simulink model "RA2"  (Simulink 8.6)
settings: Solver=ode1  StartTime=0.0  StopTime=1000  FixedStep=1/(1024*4)  RelTol=1e-3
undefined symbols (not defined in the file or in its folder): DiscIntNeverNeededParam
libraries: simulink x4
settings Model: Creator=root  LastModifiedBy=root  SimulationMode=external
settings DataIOCC: LimitDataPoints=off
settings OptimizationCC: InitFltsAndDblsToZero=on
settings DebuggingCC: SolverPrmCheckMsg=none  FcnCallInpInsideContextMsg=UseLocalSettings  UnconnectedInputMsg=none  UnconnectedOutputMsg=none  UnconnectedLineMsg=none  StrictBusMsg=Warning
settings RTWCC: SystemTargetFile=ectarget.tlc  MakeCommand="make_rtw OPTS=\"-DNETIF_ID=2\""  TemplateMakefile=ec_unix.tmf  Description=EtherCAT Real-Time Target for SOEM  RTWVerbose=off
settings GRTTargetCC: UseToolchainInfoCompliant=off  ExtMode=on

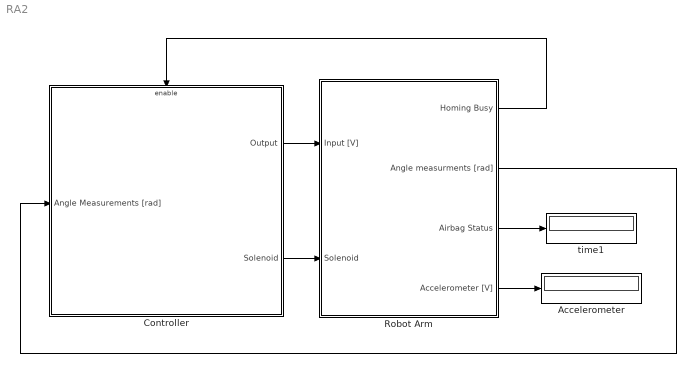
== system RA2 ==
  Accelerometer : Display
      settings: Decimation=50
  Controller : Subsystem
  Robot Arm : Subsystem
      mask help:
      | Robot Arm
      | Hardware: Brom Mechatronica
      | Software: Victor Dolk
      mask Display:
      | image(imread('RobotArm.png'))
      | color('red');port_label('output', 1, 'Homing Busy')
      | port_label('output', 2, 'Angle Measurements')
      | port_label('output', 3, 'Airbag Status')
      | port_label('output', 4, 'Accelerometer [V]')
      | port_label('input', 1, 'Input [V]')
      | port_label('input', 2, 'Solenoid')
  time1 : Display
      settings: Decimation=50
  wires:
  Controller/1(Output) -> Robot Arm/1(Input [V])
  Robot Arm/1(Homing Busy) -> Controller/Enable
  Robot Arm/2(Angle measurments [rad]) -> Controller/1(Angle Measurements [rad])
  Robot Arm/3(Airbag Status) -> time1/1
  Controller/2(Solenoid) -> Robot Arm/2(Solenoid)
  Robot Arm/4(Accelerometer [V]) -> Accelerometer/1

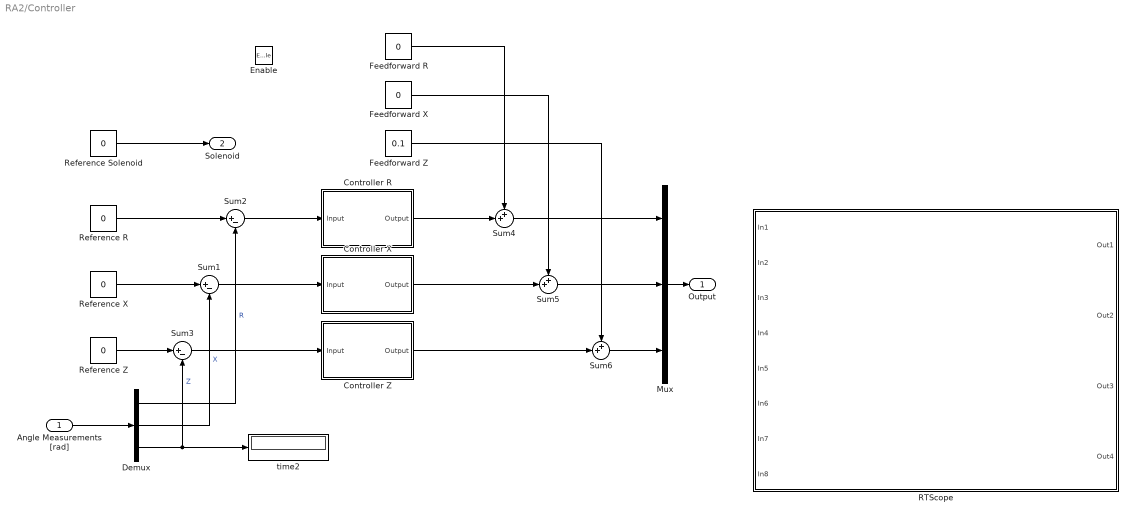
== system RA2/Controller ==
  Angle Measurements [rad] : Inport
  Enable : EnablePort
  Controller R : Subsystem
  Controller X : Subsystem
  Controller Z : Subsystem
  Demux : Demux  Outputs=3
  Feedforward R : Constant  Value=0
  Feedforward X : Constant  Value=0
  Feedforward Z : Constant  Value=0.1
  Mux : Mux  Inputs=3
  RTScope : Subsystem  mask(RTScope){}
      settings: OpenFcn=rtscope
      mask Display: image(imread('rtscope2.jpg'))
  Reference R : Constant  Value=0
  Reference Solenoid : Constant  Value=0
  Reference X : Constant  Value=0
  Reference Z : Constant  Value=0
  Sum1 : Sum  Inputs=|+-
  Sum2 : Sum  Inputs=|+-
  Sum3 : Sum  Inputs=|+-
  Sum4 : Sum  Inputs=++|  SaturateOnIntegerOverflow=on  InputSameDT=on  OutDataTypeStr=Inherit: Same as first input
  Sum5 : Sum  Inputs=++|  SaturateOnIntegerOverflow=on  InputSameDT=on  OutDataTypeStr=Inherit: Same as first input
  Sum6 : Sum  Inputs=++|  SaturateOnIntegerOverflow=on  InputSameDT=on  OutDataTypeStr=Inherit: Same as first input
  time2 : Display
      settings: Decimation=50
  Output : Outport
  Solenoid : Outport  Port=2  InitialOutput=0
  wires:
  Mux/1 -> Output/1
  Angle Measurements [rad]/1 -> Demux/1
  Sum2/1 -> Controller R/1(Input)
  Sum3/1 -> Controller Z/1(Input)
  Sum1/1 -> Controller X/1(Input)
  Demux/1 -> Sum2/2  "R"
  Demux/2 -> Sum1/2  "X"
  Demux/3 -> Sum3/2, time2/1  "Z"
  Feedforward R/1 -> Sum4/1
  Controller R/1(Output) -> Sum4/2
  Sum4/1 -> Mux/1
  Feedforward X/1 -> Sum5/1
  Controller X/1(Output) -> Sum5/2
  Sum5/1 -> Mux/2
  Controller Z/1(Output) -> Sum6/2
  Sum6/1 -> Mux/3
  Feedforward Z/1 -> Sum6/1
  Reference R/1 -> Sum2/1
  Reference X/1 -> Sum1/1
  Reference Z/1 -> Sum3/1
  Reference Solenoid/1 -> Solenoid/1

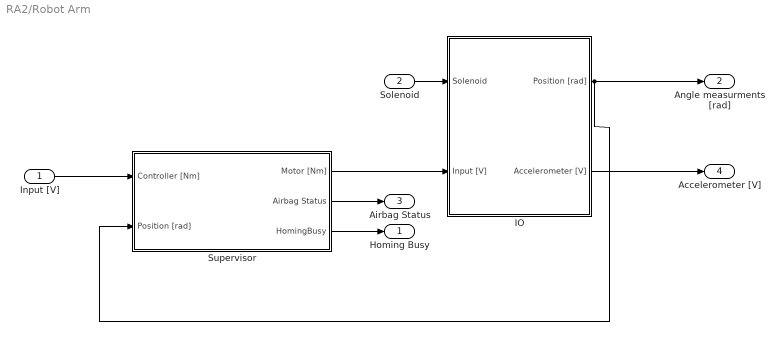
== system RA2/Robot Arm ==
  Input [V] : Inport
  Solenoid : Inport  Port=2
  IO : Subsystem
  Supervisor : Subsystem
  Homing Busy : Outport
  Angle measurments [rad] : Outport  Port=2
  Airbag Status : Outport  Port=3
  Accelerometer [V] : Outport  Port=4
  wires:
  Solenoid/1 -> IO/1(Solenoid)
  Supervisor/1(Motor [Nm]) -> IO/2(Input [V])
  Input [V]/1 -> Supervisor/1(Controller [Nm])
  IO/1(Position [rad]) -> Supervisor/2(Position [rad]), Angle measurments [rad]/1
  Supervisor/2(Airbag Status) -> Airbag Status/1
  Supervisor/3(HomingBusy) -> Homing Busy/1
  IO/2(Accelerometer [V]) -> Accelerometer [V]/1

== system RA2/Controller/Controller R ==
  Input : Inport
  Gain : Gain  Gain=0
  Output : Outport
  wires:
  Input/1 -> Gain/1
  Gain/1 -> Output/1

== system RA2/Controller/Controller X ==
  Input : Inport
  Gain : Gain  Gain=0
  Output : Outport
  wires:
  Gain/1 -> Output/1
  Input/1 -> Gain/1

== system RA2/Controller/Controller Z ==
  Input : Inport
  Gain : Gain  Gain=0
  Output : Outport
  wires:
  Input/1 -> Gain/1
  Gain/1 -> Output/1

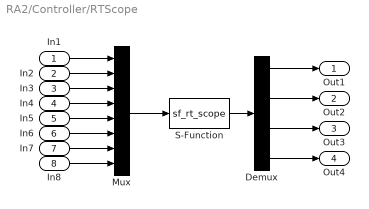
== system RA2/Controller/RTScope ==
  In1 : Inport
  In2 : Inport  Port=2
  In3 : Inport  Port=3
  In4 : Inport  Port=4
  In5 : Inport  Port=5
  In6 : Inport  Port=6
  In7 : Inport  Port=7
  In8 : Inport  Port=8
  Demux : Demux
  Mux : Mux  Inputs=8
  S-Function : S-Function  FunctionName=sf_rt_scope  Parameters=4096  SFunctionDeploymentMode=off  EnableBusSupport=off
  Out1 : Outport
  Out2 : Outport  Port=2
  Out3 : Outport  Port=3
  Out4 : Outport  Port=4
  wires:
  In8/1 -> Mux/8
  In7/1 -> Mux/7
  In6/1 -> Mux/6
  In5/1 -> Mux/5
  In4/1 -> Mux/4
  In3/1 -> Mux/3
  In2/1 -> Mux/2
  In1/1 -> Mux/1
  Demux/4 -> Out4/1
  Demux/3 -> Out3/1
  Demux/2 -> Out2/1
  Demux/1 -> Out1/1
  S-Function/1 -> Demux/1
  Mux/1 -> S-Function/1

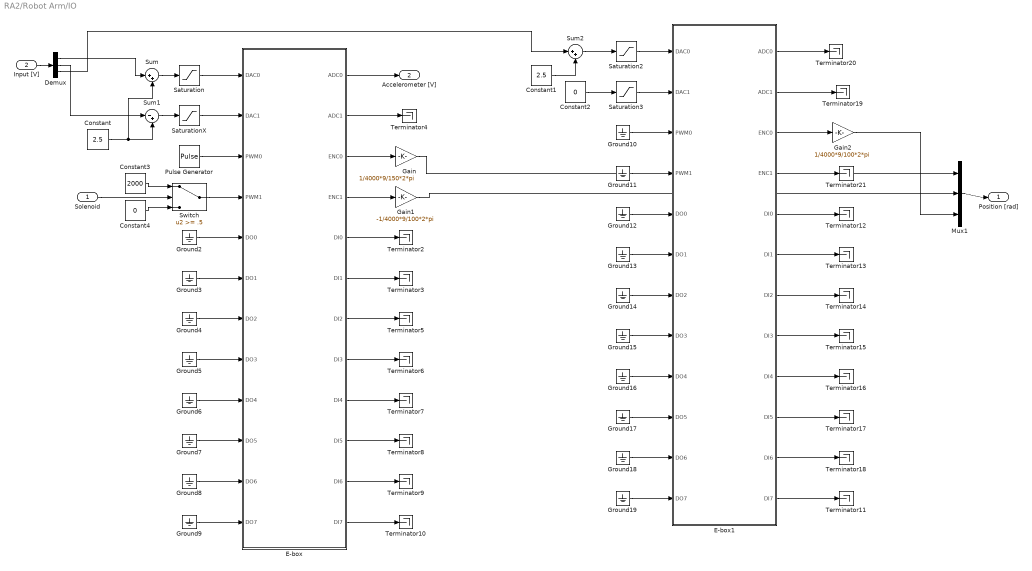
== system RA2/Robot Arm/IO ==
  Solenoid : Inport
  Input [V] : Inport  Port=2
  Constant : Constant  Value=2.5
  Constant1 : Constant  Value=2.5
  Constant2 : Constant  Value=0
  Constant3 : Constant  Value=2000
  Constant4 : Constant  Value=0
  Demux : Demux  Outputs=3
  E-box : Subsystem  mask(E-box){link_id=0}
      mask prompts: link_id "Link id (>=0)"
  E-box1 : Subsystem  mask(E-box){link_id=1}
      mask prompts: link_id "Link id (>=0)"
  Gain : Gain  Gain=1/4000*9/150*2*pi
  Gain1 : Gain  Gain=-1/4000*9/100*2*pi
  Gain2 : Gain  Gain=1/4000*9/100*2*pi
  Ground{2..19} (18 alike) : Ground
  Mux1 : Mux  Inputs=3
  Pulse Generator : DiscretePulseGenerator  PulseType=Time based  Amplitude=2000  Period=1/1024  PulseWidth=50
  Saturation : Saturate  UpperLimit=5  LowerLimit=0
  Saturation2 : Saturate  UpperLimit=5  LowerLimit=0
  Saturation3 : Saturate  UpperLimit=5  LowerLimit=0
  SaturationX : Saturate  UpperLimit=5  LowerLimit=0
  Sum : Sum  Inputs=|++
  Sum1 : Sum  Inputs=|-+
  Sum2 : Sum  Inputs=|++
  Switch : Switch  Threshold=.5
  Terminator{2..21} (20 alike) : Terminator
  Position [rad] : Outport
  Accelerometer [V] : Outport  Port=2
  wires:
  E-box/3(ENC0) -> Gain/1
  Gain/1 -> Mux1/1
  E-box1/3(ENC0) -> Gain2/1
  E-box/4(ENC1) -> Gain1/1
  Saturation/1 -> E-box/1(DAC0)
  SaturationX/1 -> E-box/2(DAC1)
  Saturation2/1 -> E-box1/1(DAC0)
  Saturation3/1 -> E-box1/2(DAC1)
  Ground2/1 -> E-box/5(DO0)
  Ground3/1 -> E-box/6(DO1)
  Ground4/1 -> E-box/7(DO2)
  Ground5/1 -> E-box/8(DO3)
  Ground6/1 -> E-box/9(DO4)
  Ground7/1 -> E-box/10(DO5)
  Ground8/1 -> E-box/11(DO6)
  Ground9/1 -> E-box/12(DO7)
  Ground10/1 -> E-box1/3(PWM0)
  Ground11/1 -> E-box1/4(PWM1)
  Ground12/1 -> E-box1/5(DO0)
  Ground13/1 -> E-box1/6(DO1)
  Ground14/1 -> E-box1/7(DO2)
  Ground15/1 -> E-box1/8(DO3)
  Ground16/1 -> E-box1/9(DO4)
  Ground17/1 -> E-box1/10(DO5)
  Ground18/1 -> E-box1/11(DO6)
  Ground19/1 -> E-box1/12(DO7)
  E-box/12(DI7) -> Terminator10/1
  E-box/11(DI6) -> Terminator9/1
  E-box/10(DI5) -> Terminator8/1
  E-box/9(DI4) -> Terminator7/1
  E-box/8(DI3) -> Terminator6/1
  E-box/7(DI2) -> Terminator5/1
  E-box/6(DI1) -> Terminator3/1
  E-box/5(DI0) -> Terminator2/1
  E-box1/12(DI7) -> Terminator11/1
  E-box1/11(DI6) -> Terminator18/1
  E-box1/10(DI5) -> Terminator17/1
  E-box1/9(DI4) -> Terminator16/1
  E-box1/8(DI3) -> Terminator15/1
  E-box1/7(DI2) -> Terminator14/1
  E-box1/6(DI1) -> Terminator13/1
  E-box1/5(DI0) -> Terminator12/1
  E-box1/2(ADC1) -> Terminator19/1
  E-box1/4(ENC1) -> Terminator21/1
  Constant2/1 -> Saturation3/1
  Gain1/1 -> Mux1/2
  Gain2/1 -> Mux1/3
  Demux/1 -> Sum/1
  Sum/1 -> Saturation/1
  Demux/2 -> Sum1/1
  Constant/1 -> Sum/2, Sum1/2
  Sum2/1 -> Saturation2/1
  Demux/3 -> Sum2/1
  Constant1/1 -> Sum2/2
  Sum1/1 -> SaturationX/1
  E-box/2(ADC1) -> Terminator4/1
  E-box1/1(ADC0) -> Terminator20/1
  Pulse Generator/1 -> E-box/3(PWM0)
  Switch/1 -> E-box/4(PWM1)
  Constant4/1 -> Switch/3
  Constant3/1 -> Switch/1
  Solenoid/1 -> Switch/2
  Input [V]/1 -> Demux/1
  Mux1/1 -> Position [rad]/1
  E-box/1(ADC0) -> Accelerometer [V]/1

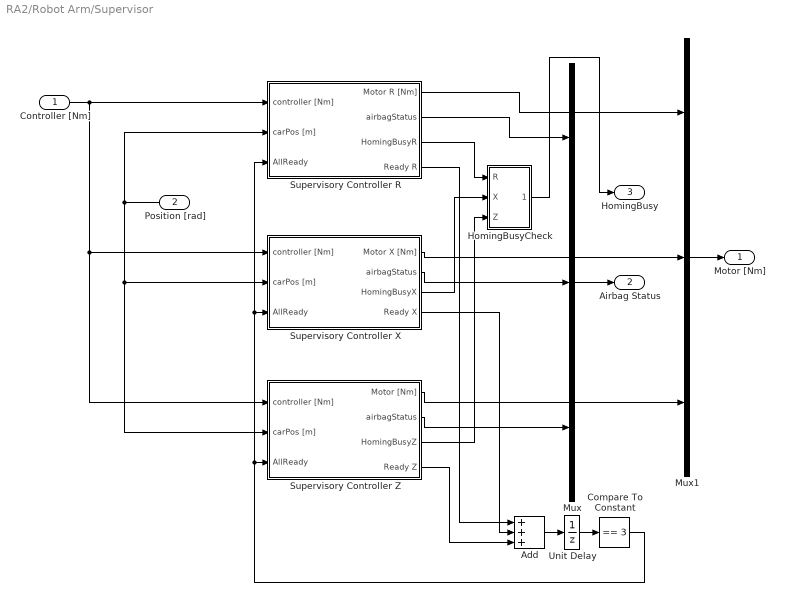
== system RA2/Robot Arm/Supervisor ==
  Controller [Nm] : Inport
  Position [rad] : Inport  Port=2
  Add : Sum  Inputs=+++
  Compare To Constant : simulink/Logic and Bit Operations/Compare To Constant  relop===  const=3  OutDataTypeStr=boolean
  HomingBusyCheck : Subsystem
  Mux : Mux  Inputs=3
  Mux1 : Mux  Inputs=3
  Supervisory Controller R : Subsystem
  Supervisory Controller X : Subsystem
  Supervisory Controller Z : Subsystem
  Unit Delay : UnitDelay  SampleTime=-1
  Motor [Nm] : Outport
  Airbag Status : Outport  Port=2
  HomingBusy : Outport  Port=3
  wires:
  Controller [Nm]/1 -> Supervisory Controller R/1(controller [Nm]), Supervisory Controller X/1(controller [Nm]), Supervisory Controller Z/1(controller [Nm])
  Mux/1 -> Airbag Status/1
  Supervisory Controller R/2(airbagStatus) -> Mux/1
  Supervisory Controller X/2(airbagStatus) -> Mux/2
  Supervisory Controller Z/2(airbagStatus) -> Mux/3
  Supervisory Controller R/1(Motor R [Nm]) -> Mux1/1
  Supervisory Controller X/1(Motor X [Nm]) -> Mux1/2
  Supervisory Controller Z/1(Motor [Nm]) -> Mux1/3
  Position [rad]/1 -> Supervisory Controller R/2(carPos [m]), Supervisory Controller X/2(carPos [m]), Supervisory Controller Z/2(carPos [m])
  Mux1/1 -> Motor [Nm]/1
  Supervisory Controller R/3(HomingBusyR) -> HomingBusyCheck/1(R)
  Supervisory Controller X/3(HomingBusyX) -> HomingBusyCheck/2(X)
  Supervisory Controller Z/3(HomingBusyZ) -> HomingBusyCheck/3(Z)
  HomingBusyCheck/1(Out1) -> HomingBusy/1
  Supervisory Controller R/4(Ready R) -> Add/1
  Supervisory Controller X/4(Ready X) -> Add/2
  Supervisory Controller Z/4(Ready Z) -> Add/3
  Compare To Constant/1 -> Supervisory Controller Z/3(AllReady), Supervisory Controller X/3(AllReady), Supervisory Controller R/3(AllReady)
  Add/1 -> Unit Delay/1
  Unit Delay/1 -> Compare To Constant/1

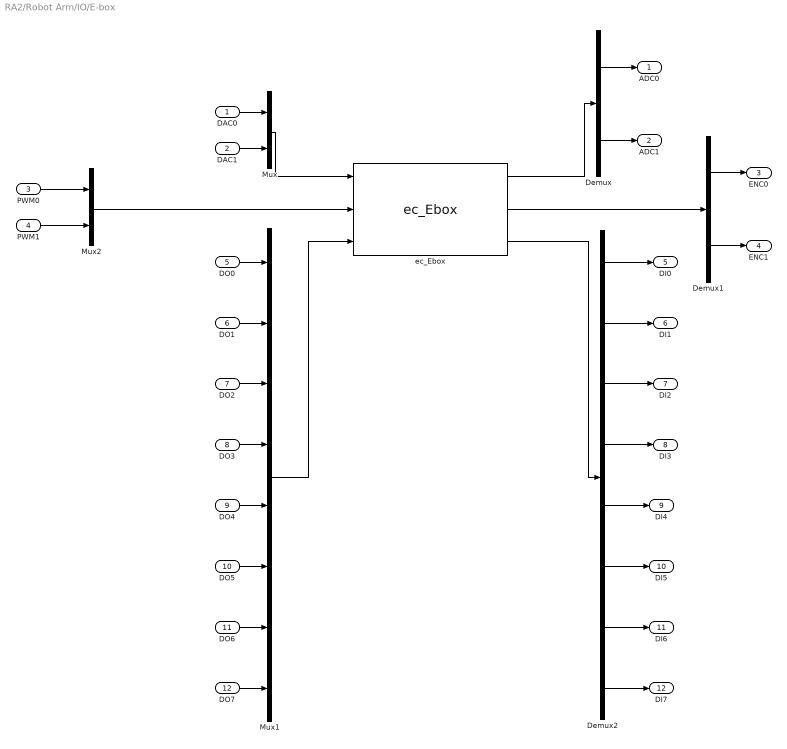
== system RA2/Robot Arm/IO/E-box ==
  DAC0 : Inport
  DAC1 : Inport  Port=2
  PWM0 : Inport  Port=3
  PWM1 : Inport  Port=4
  DO0 : Inport  Port=5
  DO1 : Inport  Port=6
  DO2 : Inport  Port=7
  DO3 : Inport  Port=8
  DO4 : Inport  Port=9
  DO5 : Inport  Port=10
  DO6 : Inport  Port=11
  DO7 : Inport  Port=12
  Demux : Demux  Outputs=2
  Demux1 : Demux  Outputs=2
  Demux2 : Demux  Outputs=8
  Mux : Mux  Inputs=2
  Mux1 : Mux  Inputs=8
  Mux2 : Mux  Inputs=2
  ec_Ebox : S-Function  FunctionName=ec_Ebox  Parameters=link_id  SFunctionDeploymentMode=off  EnableBusSupport=off  mask{link_id=link_id}
      mask prompts: link_id "analog in id (start from 1)"
      mask Display:
      | port_label('output',1,'ADC')
      | port_label('output',2,'ENC')
      | port_label('output',3,'DI')
      | port_label('input',1,'DAC')
      | port_label('input',2,'PWM')
      | port_label('input',3,'DO')
  ADC0 : Outport
  ADC1 : Outport  Port=2
  ENC0 : Outport  Port=3
  ENC1 : Outport  Port=4
  DI0 : Outport  Port=5
  DI1 : Outport  Port=6
  DI2 : Outport  Port=7
  DI3 : Outport  Port=8
  DI4 : Outport  Port=9
  DI5 : Outport  Port=10
  DI6 : Outport  Port=11
  DI7 : Outport  Port=12
  wires:
  ec_Ebox/1 -> Demux/1
  Demux/1 -> ADC0/1
  Demux/2 -> ADC1/1
  Demux1/1 -> ENC0/1
  Demux1/2 -> ENC1/1
  ec_Ebox/2 -> Demux1/1
  Mux/1 -> ec_Ebox/1
  DAC0/1 -> Mux/1
  DAC1/1 -> Mux/2
  ec_Ebox/3 -> Demux2/1
  Demux2/1 -> DI0/1
  Demux2/2 -> DI1/1
  Demux2/3 -> DI2/1
  Demux2/4 -> DI3/1
  Demux2/5 -> DI4/1
  Demux2/6 -> DI5/1
  Demux2/7 -> DI6/1
  Demux2/8 -> DI7/1
  DO0/1 -> Mux1/1
  DO1/1 -> Mux1/2
  DO2/1 -> Mux1/3
  DO3/1 -> Mux1/4
  DO4/1 -> Mux1/5
  DO5/1 -> Mux1/6
  DO6/1 -> Mux1/7
  DO7/1 -> Mux1/8
  Mux1/1 -> ec_Ebox/3
  Mux2/1 -> ec_Ebox/2
  PWM0/1 -> Mux2/1
  PWM1/1 -> Mux2/2

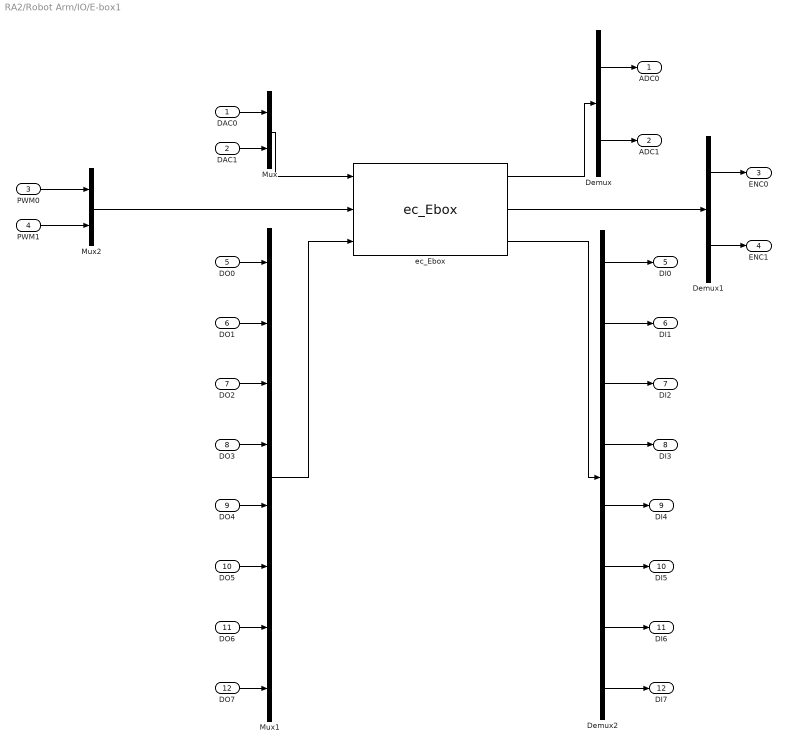
== system RA2/Robot Arm/IO/E-box1 ==
  DAC0 : Inport
  DAC1 : Inport  Port=2
  PWM0 : Inport  Port=3
  PWM1 : Inport  Port=4
  DO0 : Inport  Port=5
  DO1 : Inport  Port=6
  DO2 : Inport  Port=7
  DO3 : Inport  Port=8
  DO4 : Inport  Port=9
  DO5 : Inport  Port=10
  DO6 : Inport  Port=11
  DO7 : Inport  Port=12
  Demux : Demux  Outputs=2
  Demux1 : Demux  Outputs=2
  Demux2 : Demux  Outputs=8
  Mux : Mux  Inputs=2
  Mux1 : Mux  Inputs=8
  Mux2 : Mux  Inputs=2
  ec_Ebox : S-Function  FunctionName=ec_Ebox  Parameters=link_id  SFunctionDeploymentMode=off  EnableBusSupport=off  mask{link_id=link_id}
      mask prompts: link_id "analog in id (start from 1)"
      mask Display:
      | port_label('output',1,'ADC')
      | port_label('output',2,'ENC')
      | port_label('output',3,'DI')
      | port_label('input',1,'DAC')
      | port_label('input',2,'PWM')
      | port_label('input',3,'DO')
  ADC0 : Outport
  ADC1 : Outport  Port=2
  ENC0 : Outport  Port=3
  ENC1 : Outport  Port=4
  DI0 : Outport  Port=5
  DI1 : Outport  Port=6
  DI2 : Outport  Port=7
  DI3 : Outport  Port=8
  DI4 : Outport  Port=9
  DI5 : Outport  Port=10
  DI6 : Outport  Port=11
  DI7 : Outport  Port=12
  wires:
  PWM1/1 -> Mux2/2
  PWM0/1 -> Mux2/1
  Mux2/1 -> ec_Ebox/2
  Mux1/1 -> ec_Ebox/3
  DO7/1 -> Mux1/8
  DO6/1 -> Mux1/7
  DO5/1 -> Mux1/6
  DO4/1 -> Mux1/5
  DO3/1 -> Mux1/4
  DO2/1 -> Mux1/3
  DO1/1 -> Mux1/2
  DO0/1 -> Mux1/1
  Demux2/8 -> DI7/1
  Demux2/7 -> DI6/1
  Demux2/6 -> DI5/1
  Demux2/5 -> DI4/1
  Demux2/4 -> DI3/1
  Demux2/3 -> DI2/1
  Demux2/2 -> DI1/1
  Demux2/1 -> DI0/1
  ec_Ebox/3 -> Demux2/1
  DAC1/1 -> Mux/2
  DAC0/1 -> Mux/1
  Mux/1 -> ec_Ebox/1
  ec_Ebox/2 -> Demux1/1
  Demux1/2 -> ENC1/1
  Demux1/1 -> ENC0/1
  Demux/2 -> ADC1/1
  Demux/1 -> ADC0/1
  ec_Ebox/1 -> Demux/1

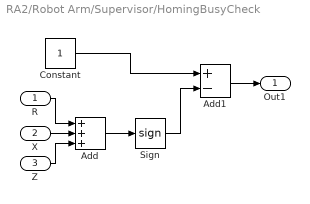
== system RA2/Robot Arm/Supervisor/HomingBusyCheck ==
  R : Inport
  X : Inport  Port=2
  Z : Inport  Port=3
  Add : Sum  Inputs=+++
  Add1 : Sum  Inputs=+-
  Constant : Constant
  Sign : Signum
  Out1 : Outport
  wires:
  Add/1 -> Sign/1
  R/1 -> Add/1
  X/1 -> Add/2
  Z/1 -> Add/3
  Constant/1 -> Add1/1
  Sign/1 -> Add1/2
  Add1/1 -> Out1/1

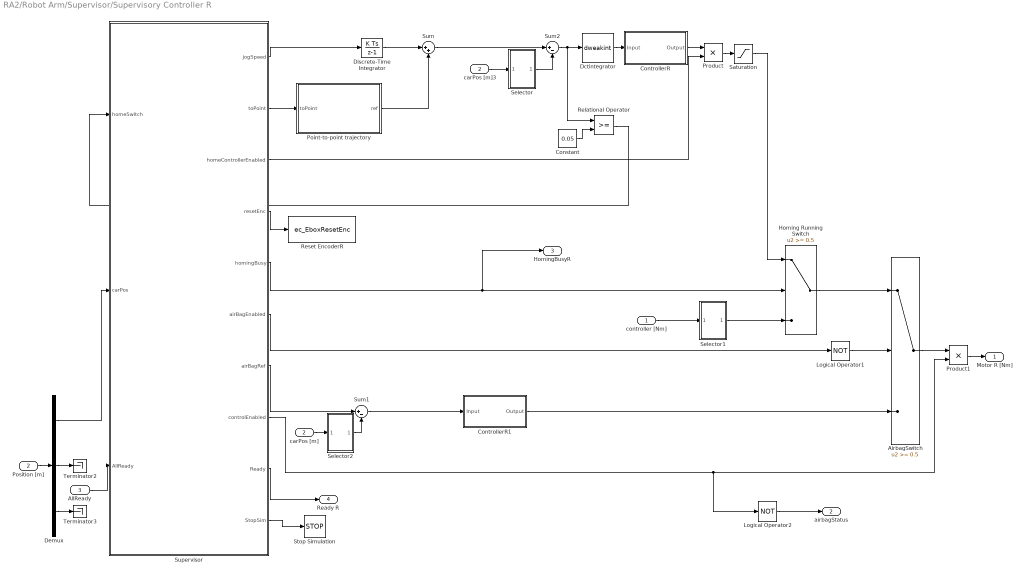
== system RA2/Robot Arm/Supervisor/Supervisory Controller R ==
  controller [Nm] : Inport
  carPos [m] : Inport  Port=2
  AllReady : Inport  Port=3
  AirbagSwitch : Switch  Threshold=0.5
  Constant : Constant  Value=0.05
  ControllerR : Subsystem  mask(Controller){Kp=60, Kv=1, notch_zeros=300, notch_damping_zeros=0.1, notch_poles=300, notch_damping_poles=0.1, roll_off_poles=120, roll_off_damping_poles=0.7}
      mask prompts: notch_zeros "Notch zeros [Hz]"; notch_damping_zeros "Notch damping zeros [-]"; notch_poles "Notch poles [Hz]"; notch_damping_poles "Notch damping poles [-]"; roll_off_poles "Roll-off poles [Hz]"; roll_off_damping_poles "Roll-off damping poles [-]"
      mask help:
      | The controller consists of three filters: a Kp/Kv, a notch and a roll-off filter.
      | You can edit the parameters below.
  ControllerR1 : Subsystem  mask(Controller){Kp=50, Kv=0.7, notch_zeros=300, notch_damping_zeros=0.1, notch_poles=300, notch_damping_poles=0.1, roll_off_poles=120, roll_off_damping_poles=0.7}
      mask prompts: notch_zeros "Notch zeros [Hz]"; notch_damping_zeros "Notch damping zeros [-]"; notch_poles "Notch poles [Hz]"; notch_damping_poles "Notch damping poles [-]"; roll_off_poles "Roll-off poles [Hz]"; roll_off_damping_poles "Roll-off damping poles [-]"
      mask help:
      | The controller consists of three filters: a Kp/Kv, a notch and a roll-off filter.
      | You can edit the parameters below.
  Dctintegrator : S-Function  FunctionName=dweakint  Parameters=[f_num 0.001]  SFunctionDeploymentMode=off  EnableBusSupport=off  mask(dctools){f_num=0.5}
      mask prompts: f_num "Zero [Hz]"
      mask help: This block implements a discrete time weak integrator filter.
      mask Display: disp('DCT integrator')
  Demux : Demux  Outputs=3
  Discrete-Time Integrator : DiscreteIntegrator  SampleTime=-1  ICPrevOutput=DiscIntNeverNeededParam  ICPrevScaledInput=DiscIntNeverNeededParam
  Homing Running Switch : Switch  Threshold=0.5
  Logical Operator1 : Logic  Operator=NOT  AllPortsSameDT=off  OutDataTypeStr=boolean
  Logical Operator2 : Logic  Operator=NOT  AllPortsSameDT=off  OutDataTypeStr=boolean
  Point-to-point trajectory : Subsystem
  Position [m] : InportShadow  Port=2
  Product : Product  RndMeth=Zero
  Product1 : Product  RndMeth=Zero
  Relational Operator : RelationalOperator  OutDataTypeStr=boolean
  Reset EncoderR : S-Function  FunctionName=ec_EboxResetEnc  Parameters=link_id, chan_id  SFunctionDeploymentMode=off  EnableBusSupport=off  mask{link_id=0, chan_id=0}
      mask prompts: link_id "Ebox ID (starting from 0)"; chan_id "Encoder channel (0 or 1)"
  Saturation : Saturate  UpperLimit=0.7  LowerLimit=-0.7
  Selector : Subsystem
  Selector1 : Subsystem
  Selector2 : Subsystem
  Stop Simulation : Stop
  Sum : Sum  Inputs=|++
  Sum1 : Sum  Inputs=|+-
  Sum2 : Sum  Inputs=|+-
  Supervisor : Stateflow chart  TreatAsAtomicUnit=on
  Terminator2 : Terminator
  Terminator3 : Terminator
  carPos [m]3 : InportShadow  Port=2
  Motor R [Nm] : Outport
  airbagStatus : Outport  Port=2
  HomingBusyR : Outport  Port=3
  Ready R : Outport  Port=4
  wires:
  Homing Running Switch/1 -> AirbagSwitch/1
  Sum2/1 -> Dctintegrator/1, Relational Operator/1
  Relational Operator/1 -> Supervisor/1(homeSwitch)
  Supervisor/1(jogSpeed) -> Discrete-Time Integrator/1
  ControllerR/1(Output) -> Product/1
  Product/1 -> Saturation/1
  Discrete-Time Integrator/1 -> Sum/1
  Point-to-point trajectory/1(ref) -> Sum/2
  Supervisor/5(homingBusy) -> Homing Running Switch/2, HomingBusyR/1
  Supervisor/3(homeControllerEnabled) -> Product/2
  Supervisor/2(toPoint) -> Point-to-point trajectory/1(toPoint)
  Supervisor/4(resetEnc) -> Reset EncoderR/1
  Supervisor/6(airBagEnabled) -> Logical Operator1/1
  Logical Operator1/1 -> AirbagSwitch/2
  Sum1/1 -> ControllerR1/1(Input)
  carPos [m]/1 -> Selector2/1(In1)
  Supervisor/7(airBagRef) -> Sum1/1
  AirbagSwitch/1 -> Product1/1
  Product1/1 -> Motor R [Nm]/1
  Supervisor/8(controlEnabled) -> Product1/2, Logical Operator2/1
  Logical Operator2/1 -> airbagStatus/1
  Sum/1 -> Sum2/1
  Position [m]/1 -> Demux/1
  Demux/1 -> Supervisor/2(carPos)
  carPos [m]3/1 -> Selector/1(In1)
  Selector/1(Out1) -> Sum2/2
  Demux/2 -> Terminator2/1
  Demux/3 -> Terminator3/1
  Selector1/1(Out1) -> Homing Running Switch/3
  controller [Nm]/1 -> Selector1/1(In1)
  Selector2/1(Out1) -> Sum1/2
  ControllerR1/1(Output) -> AirbagSwitch/3
  Constant/1 -> Relational Operator/2
  Supervisor/9(Ready) -> Ready R/1
  AllReady/1 -> Supervisor/3(AllReady)
  Supervisor/10(StopSim) -> Stop Simulation/1
  Dctintegrator/1 -> ControllerR/1(Input)
  Saturation/1 -> Homing Running Switch/1

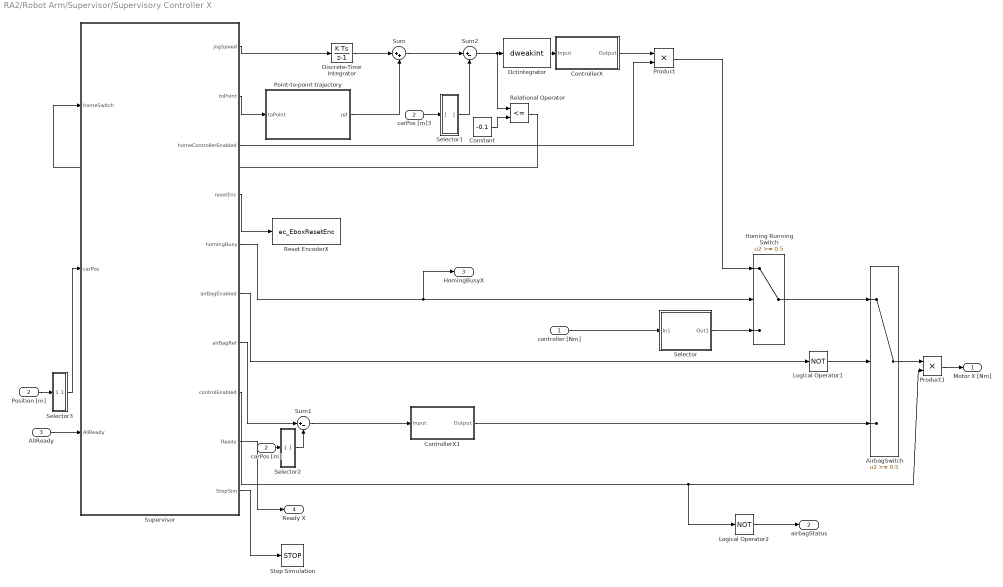
== system RA2/Robot Arm/Supervisor/Supervisory Controller X ==
  controller [Nm] : Inport
  carPos [m] : Inport  Port=2
  AllReady : Inport  Port=3
  AirbagSwitch : Switch  Threshold=0.5
  Constant : Constant  Value=-0.1
  ControllerX : Subsystem  mask(Controller){Kp=40, Kv=0.45, notch_zeros=300, notch_damping_zeros=0.1, notch_poles=300, notch_damping_poles=0.1, roll_off_poles=150, roll_off_damping_poles=0.5}
      mask prompts: notch_zeros "Notch zeros [Hz]"; notch_damping_zeros "Notch damping zeros [-]"; notch_poles "Notch poles [Hz]"; notch_damping_poles "Notch damping poles [-]"; roll_off_poles "Roll-off poles [Hz]"; roll_off_damping_poles "Roll-off damping poles [-]"
      mask help:
      | The controller consists of three filters: a Kp/Kv, a notch and a roll-off filter.
      | You can edit the parameters below.
  ControllerX1 : Subsystem  mask(Controller){Kp=40, Kv=0.45, notch_zeros=300, notch_damping_zeros=0.1, notch_poles=300, notch_damping_poles=0.1, roll_off_poles=150, roll_off_damping_poles=0.5}
      mask prompts: notch_zeros "Notch zeros [Hz]"; notch_damping_zeros "Notch damping zeros [-]"; notch_poles "Notch poles [Hz]"; notch_damping_poles "Notch damping poles [-]"; roll_off_poles "Roll-off poles [Hz]"; roll_off_damping_poles "Roll-off damping poles [-]"
      mask help:
      | The controller consists of three filters: a Kp/Kv, a notch and a roll-off filter.
      | You can edit the parameters below.
  Dctintegrator : S-Function  FunctionName=dweakint  Parameters=[f_num 0.001]  SFunctionDeploymentMode=off  EnableBusSupport=off  mask(dctools){f_num=0.5}
      mask prompts: f_num "Zero [Hz]"
      mask help: This block implements a discrete time weak integrator filter.
      mask Display: disp('DCT integrator')
  Discrete-Time Integrator : DiscreteIntegrator  SampleTime=-1  ICPrevOutput=DiscIntNeverNeededParam  ICPrevScaledInput=DiscIntNeverNeededParam
  Homing Running Switch : Switch  Threshold=0.5
  Logical Operator1 : Logic  Operator=NOT  AllPortsSameDT=off  OutDataTypeStr=boolean
  Logical Operator2 : Logic  Operator=NOT  AllPortsSameDT=off  OutDataTypeStr=boolean
  Point-to-point trajectory : Subsystem
  Position [m] : InportShadow  Port=2
  Product : Product  RndMeth=Zero
  Product1 : Product  RndMeth=Zero
  Relational Operator : RelationalOperator  Operator=<=  OutDataTypeStr=boolean
  Reset EncoderX : S-Function  FunctionName=ec_EboxResetEnc  Parameters=link_id, chan_id  SFunctionDeploymentMode=off  EnableBusSupport=off  mask{link_id=0, chan_id=1}
      mask prompts: link_id "Ebox ID (starting from 0)"; chan_id "Encoder channel (0 or 1)"
  Selector : Subsystem
  Selector1 : Subsystem
  Selector2 : Subsystem
  Selector3 : Subsystem
  Stop Simulation : Stop
  Sum : Sum  Inputs=|++
  Sum1 : Sum  Inputs=|+-
  Sum2 : Sum  Inputs=|+-
  Supervisor : Stateflow chart  TreatAsAtomicUnit=on
  carPos [m]3 : InportShadow  Port=2
  Motor X [Nm] : Outport
  airbagStatus : Outport  Port=2
  HomingBusyX : Outport  Port=3
  Ready X : Outport  Port=4
  wires:
  Position [m]/1 -> Selector3/1(In1)
  Sum/1 -> Sum2/1
  Logical Operator2/1 -> airbagStatus/1
  Supervisor/8(controlEnabled) -> Logical Operator2/1, Product1/2
  Product1/1 -> Motor X [Nm]/1
  AirbagSwitch/1 -> Product1/1
  Supervisor/7(airBagRef) -> Sum1/1
  carPos [m]/1 -> Selector2/1(In1)
  Sum1/1 -> ControllerX1/1(Input)
  Logical Operator1/1 -> AirbagSwitch/2
  Supervisor/6(airBagEnabled) -> Logical Operator1/1
  Supervisor/4(resetEnc) -> Reset EncoderX/1
  Supervisor/2(toPoint) -> Point-to-point trajectory/1(toPoint)
  Supervisor/3(homeControllerEnabled) -> Product/2
  Supervisor/5(homingBusy) -> Homing Running Switch/2, HomingBusyX/1
  Point-to-point trajectory/1(ref) -> Sum/2
  Discrete-Time Integrator/1 -> Sum/1
  Product/1 -> Homing Running Switch/1
  ControllerX/1(Output) -> Product/1
  carPos [m]3/1 -> Selector1/1(In1)
  Supervisor/1(jogSpeed) -> Discrete-Time Integrator/1
  Sum2/1 -> Dctintegrator/1, Relational Operator/1
  Homing Running Switch/1 -> AirbagSwitch/1
  controller [Nm]/1 -> Selector/1(In1)
  Selector/1(Out1) -> Homing Running Switch/3
  Selector1/1(Out1) -> Sum2/2
  Selector2/1(Out1) -> Sum1/2
  Relational Operator/1 -> Supervisor/1(homeSwitch)
  Constant/1 -> Relational Operator/2
  ControllerX1/1(Output) -> AirbagSwitch/3
  Selector3/1(Out1) -> Supervisor/2(carPos)
  AllReady/1 -> Supervisor/3(AllReady)
  Supervisor/9(Ready) -> Ready X/1
  Supervisor/10(StopSim) -> Stop Simulation/1
  Dctintegrator/1 -> ControllerX/1(Input)

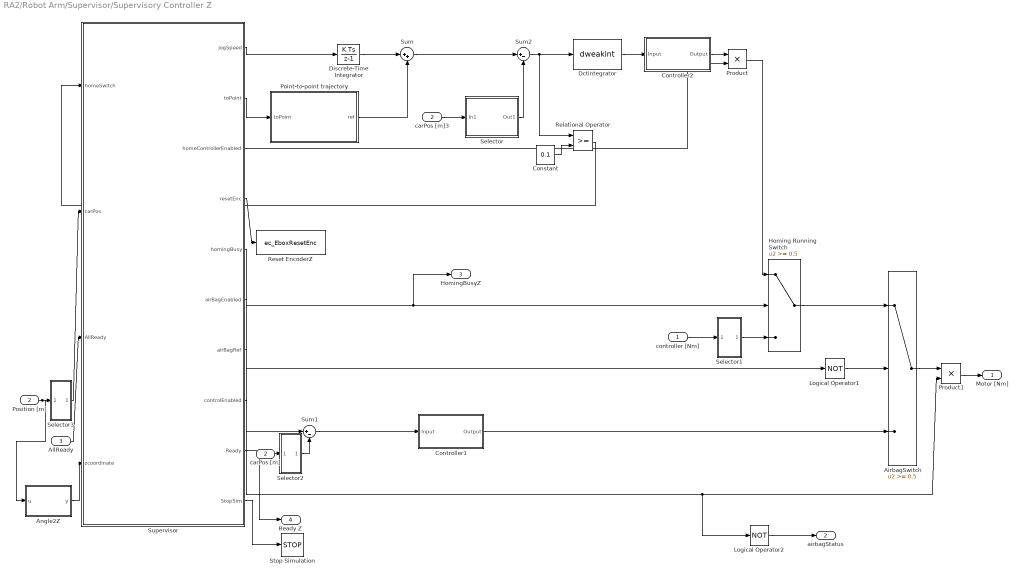
== system RA2/Robot Arm/Supervisor/Supervisory Controller Z ==
  controller [Nm] : Inport
  carPos [m] : Inport  Port=2
  AllReady : Inport  Port=3
  AirbagSwitch : Switch  Threshold=0.5
  Angle2Z : MATLAB Function  TreatAsAtomicUnit=on
  Constant : Constant  Value=0.1
  Controller1 : Subsystem  mask(Controller){Kp=75, Kv=0.5, notch_zeros=300, notch_damping_zeros=0.1, notch_poles=300, notch_damping_poles=0.1, roll_off_poles=150, roll_off_damping_poles=0.5}
      mask prompts: notch_zeros "Notch zeros [Hz]"; notch_damping_zeros "Notch damping zeros [-]"; notch_poles "Notch poles [Hz]"; notch_damping_poles "Notch damping poles [-]"; roll_off_poles "Roll-off poles [Hz]"; roll_off_damping_poles "Roll-off damping poles [-]"
      mask help:
      | The controller consists of three filters: a Kp/Kv, a notch and a roll-off filter.
      | You can edit the parameters below.
  Controller2 : Subsystem  mask(Controller){Kp=75, Kv=0.5, notch_zeros=300, notch_damping_zeros=0.1, notch_poles=300, notch_damping_poles=0.1, roll_off_poles=150, roll_off_damping_poles=0.5}
      mask prompts: notch_zeros "Notch zeros [Hz]"; notch_damping_zeros "Notch damping zeros [-]"; notch_poles "Notch poles [Hz]"; notch_damping_poles "Notch damping poles [-]"; roll_off_poles "Roll-off poles [Hz]"; roll_off_damping_poles "Roll-off damping poles [-]"
      mask help:
      | The controller consists of three filters: a Kp/Kv, a notch and a roll-off filter.
      | You can edit the parameters below.
  Dctintegrator : S-Function  FunctionName=dweakint  Parameters=[f_num 0.001]  SFunctionDeploymentMode=off  EnableBusSupport=off  mask(dctools){f_num=0.5}
      mask prompts: f_num "Zero [Hz]"
      mask help: This block implements a discrete time weak integrator filter.
      mask Display: disp('DCT integrator')
  Discrete-Time Integrator : DiscreteIntegrator  SampleTime=-1  ICPrevOutput=DiscIntNeverNeededParam  ICPrevScaledInput=DiscIntNeverNeededParam
  Homing Running Switch : Switch  Threshold=0.5
  Logical Operator1 : Logic  Operator=NOT  AllPortsSameDT=off  OutDataTypeStr=boolean
  Logical Operator2 : Logic  Operator=NOT  AllPortsSameDT=off  OutDataTypeStr=boolean
  Point-to-point trajectory : Subsystem
  Position [m] : InportShadow  Port=2
  Product : Product  RndMeth=Zero
  Product1 : Product  RndMeth=Zero
  Relational Operator : RelationalOperator  OutDataTypeStr=boolean
  Reset EncoderZ : S-Function  FunctionName=ec_EboxResetEnc  Parameters=link_id, chan_id  SFunctionDeploymentMode=off  EnableBusSupport=off  mask{link_id=1, chan_id=0}
      mask prompts: link_id "Ebox ID (starting from 0)"; chan_id "Encoder channel (0 or 1)"
  Selector : Subsystem
  Selector1 : Subsystem
  Selector2 : Subsystem
  Selector3 : Subsystem
  Stop Simulation : Stop
  Sum : Sum  Inputs=|++
  Sum1 : Sum  Inputs=|+-
  Sum2 : Sum  Inputs=|+-
  Supervisor : Stateflow chart  TreatAsAtomicUnit=on
  carPos [m]3 : InportShadow  Port=2
  Motor [Nm] : Outport
  airbagStatus : Outport  Port=2
  HomingBusyZ : Outport  Port=3
  Ready Z : Outport  Port=4
  wires:
  Homing Running Switch/1 -> AirbagSwitch/1
  Sum2/1 -> Dctintegrator/1, Relational Operator/1
  Supervisor/1(jogSpeed) -> Discrete-Time Integrator/1
  carPos [m]3/1 -> Selector/1(In1)
  controller [Nm]/1 -> Selector1/1(In1)
  Controller2/1(Output) -> Product/1
  Product/1 -> Homing Running Switch/1
  Discrete-Time Integrator/1 -> Sum/1
  Point-to-point trajectory/1(ref) -> Sum/2
  Supervisor/5(homingBusy) -> Homing Running Switch/2, HomingBusyZ/1
  Supervisor/3(homeControllerEnabled) -> Product/2
  Supervisor/2(toPoint) -> Point-to-point trajectory/1(toPoint)
  Supervisor/4(resetEnc) -> Reset EncoderZ/1
  Supervisor/6(airBagEnabled) -> Logical Operator1/1
  Logical Operator1/1 -> AirbagSwitch/2
  Sum1/1 -> Controller1/1(Input)
  carPos [m]/1 -> Selector2/1(In1)
  Supervisor/7(airBagRef) -> Sum1/1
  AirbagSwitch/1 -> Product1/1
  Product1/1 -> Motor [Nm]/1
  Supervisor/8(controlEnabled) -> Product1/2, Logical Operator2/1
  Logical Operator2/1 -> airbagStatus/1
  Position [m]/1 -> Selector3/1(In1), Angle2Z/1(u)
  Sum/1 -> Sum2/1
  Selector/1(Out1) -> Sum2/2
  Selector1/1(Out1) -> Homing Running Switch/3
  Selector2/1(Out1) -> Sum1/2
  Constant/1 -> Relational Operator/2
  Relational Operator/1 -> Supervisor/1(homeSwitch)
  Controller1/1(Output) -> AirbagSwitch/3
  Selector3/1(Out1) -> Supervisor/2(carPos)
  AllReady/1 -> Supervisor/3(AllReady)
  Supervisor/9(Ready) -> Ready Z/1
  Supervisor/10(StopSim) -> Stop Simulation/1
  Dctintegrator/1 -> Controller2/1(Input)
  Angle2Z/1(y) -> Supervisor/4(zcoordinate)

== system RA2/Robot Arm/Supervisor/Supervisory Controller R/ControllerR ==
  Input : Inport
  Dct2lowpass : S-Function  FunctionName=dlowpass2  Parameters=[f_den b_den 0.001]  SFunctionDeploymentMode=off  EnableBusSupport=off  mask(dctools){f_den=roll_off_poles, b_den=roll_off_damping_poles}
      mask prompts: f_den "Pole [Hz]"; b_den "Damping pole [-]"
      mask help: This block implements a discrete time 2nd order lowpass filter.
      mask Display: disp('DCT 2nd order lowpass')
  Dctnotch : S-Function  FunctionName=dnotch  Parameters=[f_num b_num f_den b_den 0.001]  SFunctionDeploymentMode=off  EnableBusSupport=off  mask(dctools){f_num=notch_zeros, b_num=notch_damping_zeros, f_den=notch_poles, b_den=notch_damping_poles}
      mask prompts: f_num "Zero [Hz]"; b_num "Damping zero [-]"; f_den "Pole [Hz]"; b_den "Damping pole [-]"
      mask help: This block implements a dicrete time 2nd order notch filter.
      mask Display: disp('DCT notch')
  Dctpd : S-Function  FunctionName=dpd  Parameters=[kp kv 0.001]  SFunctionDeploymentMode=off  EnableBusSupport=off  mask(dctools){kp=Kp, kv=Kv}
      mask help: This block implements a discrete time pd filter.
      mask Display: disp('DCT pd')
  Gain1 : Gain  SaturateOnIntegerOverflow=on  OutDataTypeStr=Inherit: Same as input  ParamDataTypeStr=Inherit: Same as input
  Output : Outport
  wires:
  Dct2lowpass/1 -> Output/1
  Gain1/1 -> Dctpd/1
  Input/1 -> Gain1/1
  Dctpd/1 -> Dctnotch/1
  Dctnotch/1 -> Dct2lowpass/1

== system RA2/Robot Arm/Supervisor/Supervisory Controller R/ControllerR1 ==
  Input : Inport
  Dct2lowpass : S-Function  FunctionName=dlowpass2  Parameters=[f_den b_den 0.001]  SFunctionDeploymentMode=off  EnableBusSupport=off  mask(dctools){f_den=roll_off_poles, b_den=roll_off_damping_poles}
      mask prompts: f_den "Pole [Hz]"; b_den "Damping pole [-]"
      mask help: This block implements a discrete time 2nd order lowpass filter.
      mask Display: disp('DCT 2nd order lowpass')
  Dctnotch : S-Function  FunctionName=dnotch  Parameters=[f_num b_num f_den b_den 0.001]  SFunctionDeploymentMode=off  EnableBusSupport=off  mask(dctools){f_num=notch_zeros, b_num=notch_damping_zeros, f_den=notch_poles, b_den=notch_damping_poles}
      mask prompts: f_num "Zero [Hz]"; b_num "Damping zero [-]"; f_den "Pole [Hz]"; b_den "Damping pole [-]"
      mask help: This block implements a dicrete time 2nd order notch filter.
      mask Display: disp('DCT notch')
  Dctpd : S-Function  FunctionName=dpd  Parameters=[kp kv 0.001]  SFunctionDeploymentMode=off  EnableBusSupport=off  mask(dctools){kp=Kp, kv=Kv}
      mask help: This block implements a discrete time pd filter.
      mask Display: disp('DCT pd')
  Gain1 : Gain  SaturateOnIntegerOverflow=on  OutDataTypeStr=Inherit: Same as input  ParamDataTypeStr=Inherit: Same as input
  Output : Outport
  wires:
  Input/1 -> Gain1/1
  Gain1/1 -> Dctpd/1
  Dct2lowpass/1 -> Output/1
  Dctpd/1 -> Dctnotch/1
  Dctnotch/1 -> Dct2lowpass/1

== system RA2/Robot Arm/Supervisor/Supervisory Controller R/Point-to-point trajectory ==
  toPoint : Inport
  Constant1 : Constant  Value=0
  Discrete Derivative : simulink/Discrete/Discrete Derivative  gainval=1.0  ICPrevScaledInput=0.0  InputProcessing=Inherited  OutMin=[]  OutMax=[]  OutDataType=fixdt(1, 16)  OutScaling=2^-10  DoSatur=off
  Discrete-Time Integrator : DiscreteIntegrator  InitialConditionSource=external  SampleTime=-1  ICPrevOutput=DiscIntNeverNeededParam  ICPrevScaledInput=DiscIntNeverNeededParam
  Limit Acceleration : RateLimiter  RisingSlewLimit=0.5  FallingSlewLimit=-0.5  SampleTimeMode=inherited
  Limit Speed : RateLimiter  RisingSlewLimit=0.4  FallingSlewLimit=-0.4  SampleTimeMode=inherited
  Sum : Sum  Inputs=|++
  ref : Outport
  wires:
  Sum/1 -> Limit Speed/1
  Constant1/1 -> Sum/2, Discrete-Time Integrator/2
  Limit Acceleration/1 -> Discrete-Time Integrator/1
  Discrete Derivative/1 -> Limit Acceleration/1
  Limit Speed/1 -> Discrete Derivative/1
  toPoint/1 -> Sum/1
  Discrete-Time Integrator/1 -> ref/1

== system RA2/Robot Arm/Supervisor/Supervisory Controller R/Selector ==
  In1 : Inport
  Demux1 : Demux  Outputs=3
  Terminator : Terminator
  Terminator1 : Terminator
  Out1 : Outport
  wires:
  Demux1/2 -> Terminator/1
  Demux1/3 -> Terminator1/1
  Demux1/1 -> Out1/1
  In1/1 -> Demux1/1

== system RA2/Robot Arm/Supervisor/Supervisory Controller R/Selector1 ==
  In1 : Inport
  Demux2 : Demux  Outputs=3
  Terminator4 : Terminator
  Terminator5 : Terminator
  Out1 : Outport
  wires:
  Demux2/2 -> Terminator4/1
  Demux2/3 -> Terminator5/1
  Demux2/1 -> Out1/1
  In1/1 -> Demux2/1

== system RA2/Robot Arm/Supervisor/Supervisory Controller R/Selector2 ==
  In1 : Inport
  Demux2 : Demux  Outputs=3
  Terminator4 : Terminator
  Terminator5 : Terminator
  Out1 : Outport
  wires:
  In1/1 -> Demux2/1
  Demux2/1 -> Out1/1
  Demux2/3 -> Terminator5/1
  Demux2/2 -> Terminator4/1

== system RA2/Robot Arm/Supervisor/Supervisory Controller X/ControllerX ==
  Input : Inport
  Dct2lowpass : S-Function  FunctionName=dlowpass2  Parameters=[f_den b_den 0.001]  SFunctionDeploymentMode=off  EnableBusSupport=off  mask(dctools){f_den=roll_off_poles, b_den=roll_off_damping_poles}
      mask prompts: f_den "Pole [Hz]"; b_den "Damping pole [-]"
      mask help: This block implements a discrete time 2nd order lowpass filter.
      mask Display: disp('DCT 2nd order lowpass')
  Dctnotch : S-Function  FunctionName=dnotch  Parameters=[f_num b_num f_den b_den 0.001]  SFunctionDeploymentMode=off  EnableBusSupport=off  mask(dctools){f_num=notch_zeros, b_num=notch_damping_zeros, f_den=notch_poles, b_den=notch_damping_poles}
      mask prompts: f_num "Zero [Hz]"; b_num "Damping zero [-]"; f_den "Pole [Hz]"; b_den "Damping pole [-]"
      mask help: This block implements a dicrete time 2nd order notch filter.
      mask Display: disp('DCT notch')
  Dctpd : S-Function  FunctionName=dpd  Parameters=[kp kv 0.001]  SFunctionDeploymentMode=off  EnableBusSupport=off  mask(dctools){kp=Kp, kv=Kv}
      mask help: This block implements a discrete time pd filter.
      mask Display: disp('DCT pd')
  Gain1 : Gain  SaturateOnIntegerOverflow=on  OutDataTypeStr=Inherit: Same as input  ParamDataTypeStr=Inherit: Same as input
  Output : Outport
  wires:
  Dct2lowpass/1 -> Output/1
  Gain1/1 -> Dctpd/1
  Input/1 -> Gain1/1
  Dctpd/1 -> Dctnotch/1
  Dctnotch/1 -> Dct2lowpass/1

== system RA2/Robot Arm/Supervisor/Supervisory Controller X/ControllerX1 ==
  Input : Inport
  Dct2lowpass : S-Function  FunctionName=dlowpass2  Parameters=[f_den b_den 0.001]  SFunctionDeploymentMode=off  EnableBusSupport=off  mask(dctools){f_den=roll_off_poles, b_den=roll_off_damping_poles}
      mask prompts: f_den "Pole [Hz]"; b_den "Damping pole [-]"
      mask help: This block implements a discrete time 2nd order lowpass filter.
      mask Display: disp('DCT 2nd order lowpass')
  Dctnotch : S-Function  FunctionName=dnotch  Parameters=[f_num b_num f_den b_den 0.001]  SFunctionDeploymentMode=off  EnableBusSupport=off  mask(dctools){f_num=notch_zeros, b_num=notch_damping_zeros, f_den=notch_poles, b_den=notch_damping_poles}
      mask prompts: f_num "Zero [Hz]"; b_num "Damping zero [-]"; f_den "Pole [Hz]"; b_den "Damping pole [-]"
      mask help: This block implements a dicrete time 2nd order notch filter.
      mask Display: disp('DCT notch')
  Dctpd : S-Function  FunctionName=dpd  Parameters=[kp kv 0.001]  SFunctionDeploymentMode=off  EnableBusSupport=off  mask(dctools){kp=Kp, kv=Kv}
      mask help: This block implements a discrete time pd filter.
      mask Display: disp('DCT pd')
  Gain1 : Gain  SaturateOnIntegerOverflow=on  OutDataTypeStr=Inherit: Same as input  ParamDataTypeStr=Inherit: Same as input
  Output : Outport
  wires:
  Input/1 -> Gain1/1
  Gain1/1 -> Dctpd/1
  Dct2lowpass/1 -> Output/1
  Dctpd/1 -> Dctnotch/1
  Dctnotch/1 -> Dct2lowpass/1

== system RA2/Robot Arm/Supervisor/Supervisory Controller X/Point-to-point trajectory ==
  toPoint : Inport
  Constant1 : Constant  Value=0
  Discrete Derivative : simulink/Discrete/Discrete Derivative  gainval=1.0  ICPrevScaledInput=0.0  InputProcessing=Inherited  OutMin=[]  OutMax=[]  OutDataType=fixdt(1, 16)  OutScaling=2^-10  DoSatur=off
  Discrete-Time Integrator : DiscreteIntegrator  InitialConditionSource=external  SampleTime=-1  ICPrevOutput=DiscIntNeverNeededParam  ICPrevScaledInput=DiscIntNeverNeededParam
  Limit Acceleration : RateLimiter  RisingSlewLimit=0.5  FallingSlewLimit=-0.5  SampleTimeMode=inherited
  Limit Speed : RateLimiter  RisingSlewLimit=0.4  FallingSlewLimit=-0.4  SampleTimeMode=inherited
  Sum : Sum  Inputs=|++
  ref : Outport
  wires:
  Discrete-Time Integrator/1 -> ref/1
  toPoint/1 -> Sum/1
  Limit Speed/1 -> Discrete Derivative/1
  Discrete Derivative/1 -> Limit Acceleration/1
  Limit Acceleration/1 -> Discrete-Time Integrator/1
  Constant1/1 -> Discrete-Time Integrator/2, Sum/2
  Sum/1 -> Limit Speed/1

== system RA2/Robot Arm/Supervisor/Supervisory Controller X/Selector ==
  In1 : Inport
  Demux2 : Demux  Outputs=3
  Terminator4 : Terminator
  Terminator5 : Terminator
  Out1 : Outport
  wires:
  Demux2/3 -> Terminator5/1
  Demux2/1 -> Terminator4/1
  In1/1 -> Demux2/1
  Demux2/2 -> Out1/1

== system RA2/Robot Arm/Supervisor/Supervisory Controller X/Selector1 ==
  In1 : Inport
  Demux2 : Demux  Outputs=3
  Terminator4 : Terminator
  Terminator5 : Terminator
  Out1 : Outport
  wires:
  Demux2/2 -> Out1/1
  In1/1 -> Demux2/1
  Demux2/1 -> Terminator4/1
  Demux2/3 -> Terminator5/1

== system RA2/Robot Arm/Supervisor/Supervisory Controller X/Selector2 ==
  In1 : Inport
  Demux2 : Demux  Outputs=3
  Terminator4 : Terminator
  Terminator5 : Terminator
  Out1 : Outport
  wires:
  Demux2/2 -> Out1/1
  In1/1 -> Demux2/1
  Demux2/1 -> Terminator4/1
  Demux2/3 -> Terminator5/1

== system RA2/Robot Arm/Supervisor/Supervisory Controller X/Selector3 ==
  In1 : Inport
  Demux2 : Demux  Outputs=3
  Terminator4 : Terminator
  Terminator5 : Terminator
  Out1 : Outport
  wires:
  Demux2/3 -> Terminator5/1
  Demux2/1 -> Terminator4/1
  In1/1 -> Demux2/1
  Demux2/2 -> Out1/1

== system RA2/Robot Arm/Supervisor/Supervisory Controller Z/Controller1 ==
  Input : Inport
  Dct2lowpass : S-Function  FunctionName=dlowpass2  Parameters=[f_den b_den 0.001]  SFunctionDeploymentMode=off  EnableBusSupport=off  mask(dctools){f_den=roll_off_poles, b_den=roll_off_damping_poles}
      mask prompts: f_den "Pole [Hz]"; b_den "Damping pole [-]"
      mask help: This block implements a discrete time 2nd order lowpass filter.
      mask Display: disp('DCT 2nd order lowpass')
  Dctnotch : S-Function  FunctionName=dnotch  Parameters=[f_num b_num f_den b_den 0.001]  SFunctionDeploymentMode=off  EnableBusSupport=off  mask(dctools){f_num=notch_zeros, b_num=notch_damping_zeros, f_den=notch_poles, b_den=notch_damping_poles}
      mask prompts: f_num "Zero [Hz]"; b_num "Damping zero [-]"; f_den "Pole [Hz]"; b_den "Damping pole [-]"
      mask help: This block implements a dicrete time 2nd order notch filter.
      mask Display: disp('DCT notch')
  Dctpd : S-Function  FunctionName=dpd  Parameters=[kp kv 0.001]  SFunctionDeploymentMode=off  EnableBusSupport=off  mask(dctools){kp=Kp, kv=Kv}
      mask help: This block implements a discrete time pd filter.
      mask Display: disp('DCT pd')
  Gain1 : Gain  SaturateOnIntegerOverflow=on  OutDataTypeStr=Inherit: Same as input  ParamDataTypeStr=Inherit: Same as input
  Output : Outport
  wires:
  Input/1 -> Gain1/1
  Gain1/1 -> Dctpd/1
  Dct2lowpass/1 -> Output/1
  Dctpd/1 -> Dctnotch/1
  Dctnotch/1 -> Dct2lowpass/1

== system RA2/Robot Arm/Supervisor/Supervisory Controller Z/Controller2 ==
  Input : Inport
  Dct2lowpass : S-Function  FunctionName=dlowpass2  Parameters=[f_den b_den 0.001]  SFunctionDeploymentMode=off  EnableBusSupport=off  mask(dctools){f_den=roll_off_poles, b_den=roll_off_damping_poles}
      mask prompts: f_den "Pole [Hz]"; b_den "Damping pole [-]"
      mask help: This block implements a discrete time 2nd order lowpass filter.
      mask Display: disp('DCT 2nd order lowpass')
  Dctnotch : S-Function  FunctionName=dnotch  Parameters=[f_num b_num f_den b_den 0.001]  SFunctionDeploymentMode=off  EnableBusSupport=off  mask(dctools){f_num=notch_zeros, b_num=notch_damping_zeros, f_den=notch_poles, b_den=notch_damping_poles}
      mask prompts: f_num "Zero [Hz]"; b_num "Damping zero [-]"; f_den "Pole [Hz]"; b_den "Damping pole [-]"
      mask help: This block implements a dicrete time 2nd order notch filter.
      mask Display: disp('DCT notch')
  Dctpd : S-Function  FunctionName=dpd  Parameters=[kp kv 0.001]  SFunctionDeploymentMode=off  EnableBusSupport=off  mask(dctools){kp=Kp, kv=Kv}
      mask help: This block implements a discrete time pd filter.
      mask Display: disp('DCT pd')
  Gain1 : Gain  SaturateOnIntegerOverflow=on  OutDataTypeStr=Inherit: Same as input  ParamDataTypeStr=Inherit: Same as input
  Output : Outport
  wires:
  Gain1/1 -> Dctpd/1
  Input/1 -> Gain1/1
  Dct2lowpass/1 -> Output/1
  Dctpd/1 -> Dctnotch/1
  Dctnotch/1 -> Dct2lowpass/1

== system RA2/Robot Arm/Supervisor/Supervisory Controller Z/Point-to-point trajectory ==
  toPoint : Inport
  Constant1 : Constant  Value=0
  Discrete Derivative : simulink/Discrete/Discrete Derivative  gainval=1.0  ICPrevScaledInput=0.0  InputProcessing=Inherited  OutMin=[]  OutMax=[]  OutDataType=fixdt(1, 16)  OutScaling=2^-10  DoSatur=off
  Discrete-Time Integrator : DiscreteIntegrator  InitialConditionSource=external  SampleTime=-1  ICPrevOutput=DiscIntNeverNeededParam  ICPrevScaledInput=DiscIntNeverNeededParam
  Limit Acceleration : RateLimiter  RisingSlewLimit=0.5  FallingSlewLimit=-0.5  SampleTimeMode=inherited
  Limit Speed : RateLimiter  RisingSlewLimit=0.2  FallingSlewLimit=-0.2  SampleTimeMode=inherited
  Sum : Sum  Inputs=|++
  ref : Outport
  wires:
  Sum/1 -> Limit Speed/1
  Constant1/1 -> Sum/2, Discrete-Time Integrator/2
  Limit Acceleration/1 -> Discrete-Time Integrator/1
  Discrete Derivative/1 -> Limit Acceleration/1
  Limit Speed/1 -> Discrete Derivative/1
  toPoint/1 -> Sum/1
  Discrete-Time Integrator/1 -> ref/1

== system RA2/Robot Arm/Supervisor/Supervisory Controller Z/Selector ==
  In1 : Inport
  Demux2 : Demux  Outputs=3
  Terminator4 : Terminator
  Terminator5 : Terminator
  Out1 : Outport
  wires:
  Demux2/1 -> Terminator4/1
  In1/1 -> Demux2/1
  Demux2/2 -> Terminator5/1
  Demux2/3 -> Out1/1

== system RA2/Robot Arm/Supervisor/Supervisory Controller Z/Selector1 ==
  In1 : Inport
  Demux2 : Demux  Outputs=3
  Terminator4 : Terminator
  Terminator5 : Terminator
  Out1 : Outport
  wires:
  Demux2/3 -> Out1/1
  Demux2/2 -> Terminator5/1
  In1/1 -> Demux2/1
  Demux2/1 -> Terminator4/1

== system RA2/Robot Arm/Supervisor/Supervisory Controller Z/Selector2 ==
  In1 : Inport
  Demux2 : Demux  Outputs=3
  Terminator4 : Terminator
  Terminator5 : Terminator
  Out1 : Outport
  wires:
  Demux2/1 -> Terminator4/1
  In1/1 -> Demux2/1
  Demux2/2 -> Terminator5/1
  Demux2/3 -> Out1/1

== system RA2/Robot Arm/Supervisor/Supervisory Controller Z/Selector3 ==
  In1 : Inport
  Demux2 : Demux  Outputs=3
  Terminator4 : Terminator
  Terminator5 : Terminator
  Out1 : Outport
  wires:
  Demux2/3 -> Out1/1
  Demux2/2 -> Terminator5/1
  In1/1 -> Demux2/1
  Demux2/1 -> Terminator4/1

== matlab function Robot Arm/Supervisor/Supervisory Controller Z/Angle2Z ==
  data: u input double; y output double
function y = fcn(u)

initialanglex = pi/2;
initialanglez = (25.0/180)*pi;
thetax = -u(2)+initialanglex;
thetaz = u(3)+initialanglez;

theta1 = thetax;
theta2 = thetaz;

% parameters

l1 = 80e-3;
l2 = 130e-3;
l3 = 165e-3;
l4 = 130e-3;
l5 = 120e-3;
l6 = 120e-3 + 65e-3;

% functions

fx1 = l1*cos(theta1);
fy1 = l1*sin(theta1);

fx2 = l2*cos(theta2);
fy2 = l3 + l2*sin(theta2);

d12 = sqrt((fx2 - fx1)^2 + (fy2 - fy1)^2);
d13 = sqrt(fx1^2 + (l3 - fy1)^2);

phi1 = acos((l2^2 + d12^2 -d13^2)/(2*d12*l2));
phi2 = acos((l5^2 + d12^2 -l4^2)/(2*d12*l5));

yf = fy2- l6*sin(pi - phi1 - phi2 - theta2);

y = yf-13e-3;

== stateflow chart Robot Arm/Supervisor/Supervisory Controller R/Supervisor ==
  state Homing
    entry:
    %Set jog speed and homing state
    Ready=0;
    toPoint = 0;
    homingBusy = 1;
    jogSpeed = 0.4;
    homeControllerEnabled=1;
  state MovetoX0
    entry:
    jogSpeed = 0.0;
    toPoint = -2.15
  state ResetEnc
    entry:
    resetEnc=1;
    homeControllerEnabled=0;
  state DisableOutputs
    entry:
    controlEnabled=0;
    StopSim=1;
  state EnableRunAndSafety
    entry:
    resetEnc=0;
    homingBusy=0;
  state AirbagLeft
    entry:
    airBagEnabled = 1;
    airBagRef=-1.4;
  state AirbagRight
    entry:
    airBagEnabled = 1;
    airBagRef=1.4;
  state WaitForRest
    Ready = 1;
  state CheckRobotIsON
  state STOPRobotIsOFF
    entry:
    StopSim=1;
  state RobotIsON
  (default) -> Homing
  AirbagLeft -> DisableOutputs : after(5,sec)
  AirbagRight -> DisableOutputs : after(5,sec)
  EnableRunAndSafety -> AirbagLeft [order 1] : [carPos<-1.4]
  Homing -> MovetoX0 : %Transition if homeswitch becomes high
      | [homeSwitch]
  EnableRunAndSafety -> AirbagRight [order 2] : [carPos>1.4]
  MovetoX0 -> CheckRobotIsON : %Allow time for moving
      | after(0.5,sec)
  CheckRobotIsON -> STOPRobotIsOFF [order 1] : [carPos<0.1]
  CheckRobotIsON -> RobotIsON [order 2]
  RobotIsON -> WaitForRest : after(9,sec)
  ResetEnc -> EnableRunAndSafety : after(0.01,sec)
  WaitForRest -> ResetEnc : [AllReady]
  data: jogSpeed output double; toPoint output double; homeControllerEnabled output double; resetEnc output double; homingBusy output double =1; homeSwitch input boolean; carPos input double; airBagEnabled output double =0; airBagRef output double =0; controlEnabled output double =1; Ready output double =1; AllReady input boolean; StopSim output double =0

== stateflow chart Robot Arm/Supervisor/Supervisory Controller X/Supervisor ==
  state Homing
    entry:
    %Set jog speed and homing state
    jogSpeed = -0.2;
    homeControllerEnabled=1;
  state MovetoX0
    entry:
    jogSpeed = 0.0;
    toPoint = 0.7854-0.355-0.0595428;
  state ResetEnc
    entry:
    resetEnc=1;
    homeControllerEnabled=0;
  state DisableOutputs
    entry:
    controlEnabled=0;
    StopSim=1;
  state EnableRunAndSafety
    entry:
    resetEnc=0;
    homingBusy=0;
  state AirbagLeft
    entry:
    airBagEnabled = 1;
    airBagRef=-0.1;
  state AirbagRight
    entry:
    airBagEnabled = 1;
    airBagRef=1.13;
  state WaitForZ
    entry:
    toPoint = 0;
    Ready = 0;
    homingBusy = 1;
    jogSpeed=0.0;
  state WaitForRest
    Ready = 1;
  AirbagLeft -> DisableOutputs : after(5,sec)
  (default) -> WaitForZ
  AirbagRight -> DisableOutputs : after(5,sec)
  EnableRunAndSafety -> AirbagLeft [order 1] : [carPos<-0.1]
  WaitForZ -> Homing : after(3,sec)
  EnableRunAndSafety -> AirbagRight [order 2] : [carPos>1.15 ]
  Homing -> MovetoX0 : %Transition if homeswitch becomes high
      | [homeSwitch]
  MovetoX0 -> WaitForRest : %Allow time for moving
      | after(7,sec)
  ResetEnc -> EnableRunAndSafety : after(0.01,sec)
  WaitForRest -> ResetEnc : [AllReady]
  data: jogSpeed output double; toPoint output double; homeControllerEnabled output double; resetEnc output double; homingBusy output double =1; homeSwitch input boolean; carPos input double; airBagEnabled output double =0; airBagRef output double =0; controlEnabled output double =1; Ready output double =1; AllReady input boolean; StopSim output double =0

== stateflow chart Robot Arm/Supervisor/Supervisory Controller Z/Supervisor ==
  state Homing
    entry:
    %Set jog speed and homing state
    toPoint = 0;
    Ready = 0;
    homingBusy = 1;
    jogSpeed = 0.2;
    homeControllerEnabled=1;
  state MovetoX0
    entry:
    jogSpeed = 0.0;
    toPoint =-0.7854;
  state ResetEnc
    entry:
    resetEnc=1;
    homeControllerEnabled=0;
    Ready = 1;
  state DisableOutputs
    entry:
    controlEnabled=0;
    StopSim=1;
  state EnableRunAndSafety
    entry:
    resetEnc=0;
    homingBusy=0;
  state AirbagLeft
    entry:
    currentcarPos = carPos;
    airBagEnabled = 1;
    airBagRef=currentcarPos+0.02
  state AirbagRight
    entry:
    airBagEnabled = 1;
    airBagRef=0.48;
  state WaitForRest
    Ready = 1;
  (default) -> Homing
  AirbagLeft -> DisableOutputs : after(5,sec)
  AirbagRight -> DisableOutputs : after(5,sec)
  Homing -> MovetoX0 : %Transition if homeswitch becomes high
      | [homeSwitch]
  EnableRunAndSafety -> AirbagLeft [order 1] : [zcoordinate<-0.0225]
  EnableRunAndSafety -> AirbagRight [order 2] : [carPos>0.5]
  MovetoX0 -> WaitForRest : %Allow time for moving
      | after(7,sec)
  ResetEnc -> EnableRunAndSafety : after(0.01,sec)
  WaitForRest -> ResetEnc : [AllReady]
  data: jogSpeed output double; toPoint output double; homeControllerEnabled output double; resetEnc output double; homingBusy output double =1; homeSwitch input boolean; carPos input double; airBagEnabled output double =0; airBagRef output double =0; controlEnabled output double =1; Ready output double =1; AllReady input boolean; StopSim output double =0; zcoordinate input double; currentcarPos local double
